simulink model "HVDCVSCBased"  (R2024b)
settings: Solver=ode45  StartTime=0.0  StopTime=3  FixedStep=Ts_Power  RelTol=1e-3  AbsTol=1e-2
InitFcn:
  | Fnom = 50;        % Hz
  | 
  | Fc = 27*Fnom;   % (Hz)
  | Ts_Power = 1/(Fc*100);
  | Ts_Control = Ts_Power*10;
undefined symbols (not defined in the file or in its folder): D1, Delta, DiscIntNeverNeededParam, magnitude
libraries: spsSecondOrderFilterLib x20, spsSeriesRLCBranchLib x14, spsMeanVariableFrequencyLib x12, spsabctoAlphaBetaZeroLib x8, spsThreePhaseVIMeasurementLib x6, spsAlphaBetaZerotodq0Lib x6, spsCurrentMeasurementLib x4, spsThreePhaseHarmonicFilterLib x4, spsVoltageMeasurementLib x4, spsFirstOrderFilterLib x4, spsGroundLib x3, spsThreePhaseSeriesRLCBranchLib x3
(part 5 of 5)

== system HVDCVSCBased/VSC Controller Station 1/Discrete VSC Controller /Outer Active-Reactive Power and Voltage Loop/Active_Power_Control/Ramping/Rate Limiter with external rates & reset (discrete) IC:0 ==
  note: Rate Limiter with external rates & reset (Discrete)
  note: IC=ic
  note: Max= 4
      | Min =1
  note: Silvano Casoria
      | IREQ
  In : Inport
  up_rate : Inport  Port=2
  down_rate : Inport  Port=3
  R : Inport  Port=4
  Abs : Abs
  Constant3 : Constant
  Data Type Conversion1 : DataTypeConversion
  Data Type Conversion2 : DataTypeConversion
  Data Type Conversion3 : DataTypeConversion
  Gain1 : Gain  Gain=2  SaturateOnIntegerOverflow=on  OutDataTypeStr=Inherit: Same as input  ParamDataTypeStr=Inherit: Same as input
  Gain2 : Gain  Gain=3  SaturateOnIntegerOverflow=on  OutDataTypeStr=Inherit: Same as input  ParamDataTypeStr=Inherit: Same as input
  Gain3 : Gain  Gain=st  SaturateOnIntegerOverflow=on  OutDataTypeStr=Inherit: Same as input  ParamDataTypeStr=Inherit: Same as input
  Gain4 : Gain  Gain=-st  SaturateOnIntegerOverflow=on  OutDataTypeStr=Inherit: Same as input  ParamDataTypeStr=Inherit: Same as input
  Multiport Switch : MultiPortSwitch  Inputs=4
  Relational Operator : RelationalOperator  Operator=>
  Relational Operator2 : RelationalOperator  Operator=<
  Saturation : Saturate  UpperLimit=4  LowerLimit=1
  Sum : Sum  Inputs=+-  InputSameDT=on  SaturateOnIntegerOverflow=on  OutDataTypeStr=Inherit: Same as first input
  Sum1 : Sum  Inputs=++++  InputSameDT=on  SaturateOnIntegerOverflow=on  OutDataTypeStr=Inherit: Same as first input
  Sum2 : Sum  InputSameDT=on  SaturateOnIntegerOverflow=on  OutDataTypeStr=Inherit: Same as first input
  Sum3 : Sum  InputSameDT=on  SaturateOnIntegerOverflow=on  OutDataTypeStr=Inherit: Same as first input
  Unit Delay : UnitDelay  InitialCondition=ic  SampleTime=st  HasFrameUpgradeWarning=on
  " " : Outport  InitialOutput=0  VectorParamsAs1DForOutWhenUnconnected=off
  wires:
  Gain2/1 -> Sum1/3
  Constant3/1 -> Sum1/4
  Relational Operator/1 -> Data Type Conversion2/1
  Gain1/1 -> Sum1/2
  Saturation/1 -> Multiport Switch/1
  Sum1/1 -> Saturation/1
  R/1 -> Data Type Conversion3/1
  Sum3/1 -> Multiport Switch/4
  Sum2/1 -> Multiport Switch/3
  In/1 -> Multiport Switch/5, Multiport Switch/2, Sum/1
  Relational Operator2/1 -> Data Type Conversion1/1
  Sum/1 -> Relational Operator2/1, Relational Operator/1  "Rate"
  Multiport Switch/1 -> " "/1, Unit Delay/1
  Gain4/1 -> Sum3/2, Relational Operator2/2
  Gain3/1 -> Sum2/2, Relational Operator/2
  Unit Delay/1 -> Sum3/1, Sum2/1, Sum/2
  up_rate/1 -> Gain3/1
  down_rate/1 -> Abs/1
  Abs/1 -> Gain4/1
  Data Type Conversion1/1 -> Gain1/1
  Data Type Conversion2/1 -> Sum1/1
  Data Type Conversion3/1 -> Gain2/1

== system HVDCVSCBased/VSC Controller Station 2/Discrete VSC Controller /Outer Active-Reactive Power and Voltage Loop/Active_Power_Control/Ramping/Rate Limiter with external rates & reset (discrete) IC:0 ==
  note: Rate Limiter with external rates & reset (Discrete)
  note: IC=ic
  note: Max= 4
      | Min =1
  note: Silvano Casoria
      | IREQ
  In : Inport
  up_rate : Inport  Port=2
  down_rate : Inport  Port=3
  R : Inport  Port=4
  Abs : Abs
  Constant3 : Constant
  Data Type Conversion1 : DataTypeConversion
  Data Type Conversion2 : DataTypeConversion
  Data Type Conversion3 : DataTypeConversion
  Gain1 : Gain  Gain=2  SaturateOnIntegerOverflow=on  OutDataTypeStr=Inherit: Same as input  ParamDataTypeStr=Inherit: Same as input
  Gain2 : Gain  Gain=3  SaturateOnIntegerOverflow=on  OutDataTypeStr=Inherit: Same as input  ParamDataTypeStr=Inherit: Same as input
  Gain3 : Gain  Gain=st  SaturateOnIntegerOverflow=on  OutDataTypeStr=Inherit: Same as input  ParamDataTypeStr=Inherit: Same as input
  Gain4 : Gain  Gain=-st  SaturateOnIntegerOverflow=on  OutDataTypeStr=Inherit: Same as input  ParamDataTypeStr=Inherit: Same as input
  Multiport Switch : MultiPortSwitch  Inputs=4
  Relational Operator : RelationalOperator  Operator=>
  Relational Operator2 : RelationalOperator  Operator=<
  Saturation : Saturate  UpperLimit=4  LowerLimit=1
  Sum : Sum  Inputs=+-  InputSameDT=on  SaturateOnIntegerOverflow=on  OutDataTypeStr=Inherit: Same as first input
  Sum1 : Sum  Inputs=++++  InputSameDT=on  SaturateOnIntegerOverflow=on  OutDataTypeStr=Inherit: Same as first input
  Sum2 : Sum  InputSameDT=on  SaturateOnIntegerOverflow=on  OutDataTypeStr=Inherit: Same as first input
  Sum3 : Sum  InputSameDT=on  SaturateOnIntegerOverflow=on  OutDataTypeStr=Inherit: Same as first input
  Unit Delay : UnitDelay  InitialCondition=ic  SampleTime=st  HasFrameUpgradeWarning=on
  " " : Outport  InitialOutput=0  VectorParamsAs1DForOutWhenUnconnected=off
  wires:
  Gain2/1 -> Sum1/3
  Constant3/1 -> Sum1/4
  Relational Operator/1 -> Data Type Conversion2/1
  Gain1/1 -> Sum1/2
  Saturation/1 -> Multiport Switch/1
  Sum1/1 -> Saturation/1
  R/1 -> Data Type Conversion3/1
  Sum3/1 -> Multiport Switch/4
  Sum2/1 -> Multiport Switch/3
  In/1 -> Multiport Switch/5, Multiport Switch/2, Sum/1
  Relational Operator2/1 -> Data Type Conversion1/1
  Sum/1 -> Relational Operator2/1, Relational Operator/1  "Rate"
  Multiport Switch/1 -> " "/1, Unit Delay/1
  Gain4/1 -> Sum3/2, Relational Operator2/2
  Gain3/1 -> Sum2/2, Relational Operator/2
  Unit Delay/1 -> Sum3/1, Sum2/1, Sum/2
  up_rate/1 -> Gain3/1
  down_rate/1 -> Abs/1
  Abs/1 -> Gain4/1
  Data Type Conversion1/1 -> Gain1/1
  Data Type Conversion2/1 -> Sum1/1
  Data Type Conversion3/1 -> Gain2/1
